simulink model "System"  (R2019b)
settings: Solver=VariableStepAuto  StartTime=0.0  StopTime=10.0  RelTol=1e-3
PreLoadFcn:
  | load AllBuses
settings Model: Creator=visha  LastModifiedBy=visha
settings OptimizationCC: DefaultParameterBehavior=Inlined

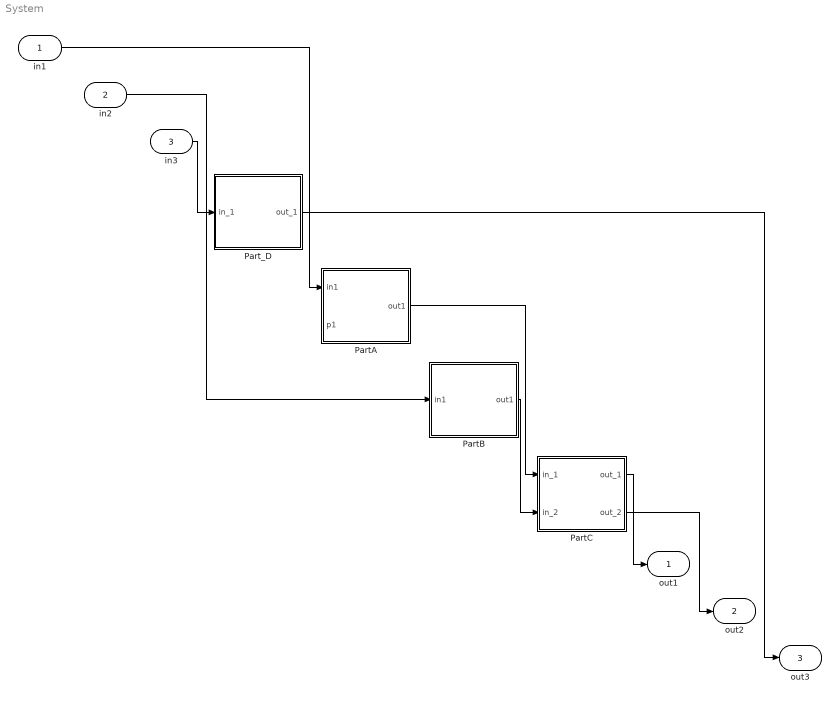
== system System ==
  in1 : Inport  OutDataTypeStr=Bus: Bus_1  BusOutputAsStruct=on
  in2 : Inport  Port=2  OutDataTypeStr=int32
  in3 : Inport  Port=3  OutDataTypeStr=Bus: Bus_2  BusOutputAsStruct=on
  PartA : Subsystem
  PartB : Subsystem
  PartC : Subsystem
  Part_D : Subsystem
  out1 : Outport  OutDataTypeStr=double
  out2 : Outport  Port=2  OutDataTypeStr=boolean
  out3 : Outport  Port=3  OutDataTypeStr=Bus: Bus_3  BusOutputAsStruct=on
  wires:
  in1/1 -> PartA/1(in1)
  in2/1 -> PartB/1(in1)
  Part_D/1(out_1) -> out3/1
  PartA/1(out1) -> PartC/1(in_1)
  PartB/1(out1) -> PartC/2(in_2)
  PartC/1(out_1) -> out1/1
  PartC/2(out_2) -> out2/1
  in3/1 -> Part_D/1(in_1)

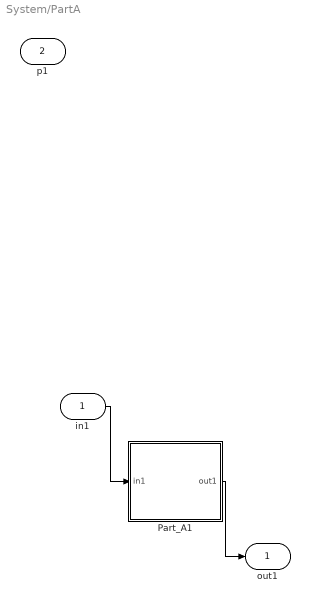
== system System/PartA ==
  in1 : Inport  BusOutputAsStruct=on
  p1 : Inport  Port=2  OutDataTypeStr=boolean
  Part_A1 : Subsystem
  out1 : Outport  OutDataTypeStr=double
  wires:
  in1/1 -> Part_A1/1(in1)
  Part_A1/1(out1) -> out1/1

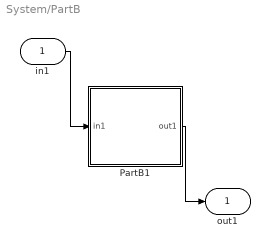
== system System/PartB ==
  in1 : Inport  OutDataTypeStr=int32
  PartB1 : Subsystem
  out1 : Outport  OutDataTypeStr=int32
  wires:
  in1/1 -> PartB1/1(in1)
  PartB1/1(out1) -> out1/1

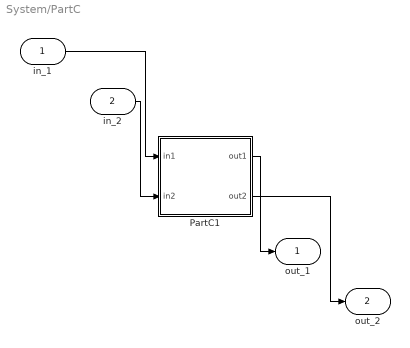
== system System/PartC ==
  in_1 : Inport  OutDataTypeStr=double
  in_2 : Inport  Port=2  OutDataTypeStr=int32
  PartC1 : Subsystem
  out_1 : Outport  OutDataTypeStr=double
  out_2 : Outport  Port=2  OutDataTypeStr=boolean
  wires:
  in_1/1 -> PartC1/1(in1)
  in_2/1 -> PartC1/2(in2)
  PartC1/1(out1) -> out_1/1
  PartC1/2(out2) -> out_2/1

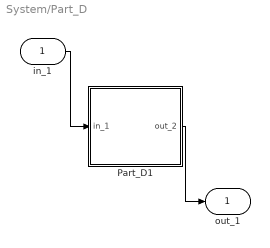
== system System/Part_D ==
  in_1 : Inport  OutDataTypeStr=Bus: Bus_2  BusOutputAsStruct=on
  Part_D1 : Subsystem
  out_1 : Outport  OutDataTypeStr=Bus: Bus_3  BusOutputAsStruct=on
  wires:
  in_1/1 -> Part_D1/1(in_1)
  Part_D1/1(out_2) -> out_1/1

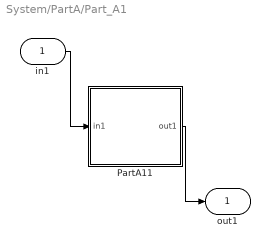
== system System/PartA/Part_A1 ==
  in1 : Inport  OutDataTypeStr=Bus: Bus_1  BusOutputAsStruct=on
  PartA11 : Subsystem
  out1 : Outport  OutDataTypeStr=double
  wires:
  PartA11/1(out1) -> out1/1
  in1/1 -> PartA11/1(in1)

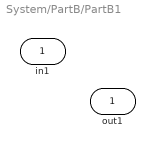
== system System/PartB/PartB1 ==
  in1 : Inport  OutDataTypeStr=int32
  out1 : Outport  OutDataTypeStr=int32

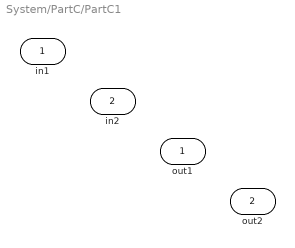
== system System/PartC/PartC1 ==
  in1 : Inport  OutDataTypeStr=double
  in2 : Inport  Port=2  OutDataTypeStr=int32
  out1 : Outport  OutDataTypeStr=double
  out2 : Outport  Port=2  OutDataTypeStr=boolean

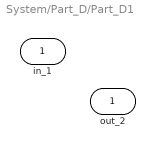
== system System/Part_D/Part_D1 ==
  in_1 : Inport  OutDataTypeStr=Bus: Bus_2  BusOutputAsStruct=on
  out_2 : Outport  OutDataTypeStr=Bus: Bus_3  BusOutputAsStruct=on

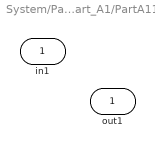
== system System/PartA/Part_A1/PartA11 ==
  in1 : Inport  OutDataTypeStr=Bus: Bus_1  BusOutputAsStruct=on
  out1 : Outport  OutDataTypeStr=double
